simulink model "MOT_CTRL_PWM_FUN_002"  (R2025a)
settings: Solver=FixedStepAuto  StartTime=0.0  StopTime=10.0  FixedStep=1e-4  RelTol=1e-3
settings Model: DataDictionary=PwmGenerator.sldd  Creator=tecnicomcbti  LastModifiedBy=tecnicomcbti

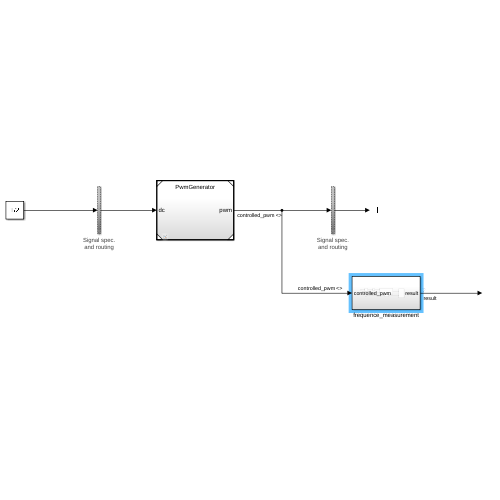
[thumbnail: Simulink's stored preview of the top-level diagram]
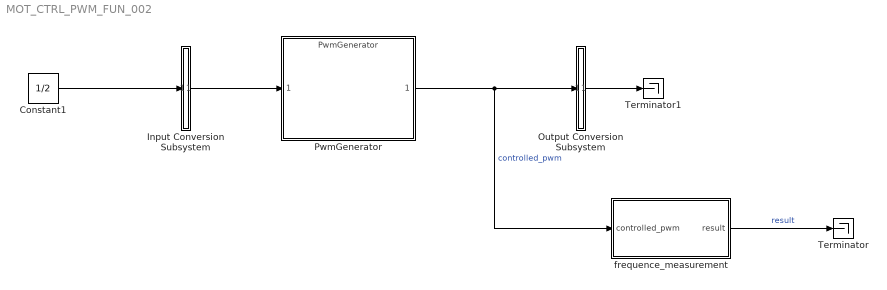
== system MOT_CTRL_PWM_FUN_002 ==
  Constant1 : Constant  Value=1/2
  Input Conversion Subsystem : Subsystem  Tag=__SLT_ICS__  Description=|
      | Signal spec.
      | and routing
      settings: AttributesFormatString=%<Description>
  Output Conversion Subsystem : Subsystem  Tag=__SLT_OCS__  Description=|
      | Signal spec.
      | and routing
      settings: AttributesFormatString=%<Description>
  PwmGenerator : ModelReference  ModelNameDialog=PwmGenerator  SimulationMode=Normal  ModelReferenceVersion=1.9
  Terminator : Terminator
  Terminator1 : Terminator
  frequence_measurement : Subsystem
  wires:
  Constant1/1 -> Input Conversion Subsystem/1(Inport_1)
  Input Conversion Subsystem/1(Outport_1) -> PwmGenerator/1
  PwmGenerator/1 -> frequence_measurement/1(controlled_pwm), Output Conversion Subsystem/1(Inport_1)  "controlled_pwm"
  frequence_measurement/1(result) -> Terminator/1  "result"
  Output Conversion Subsystem/1(Outport_1) -> Terminator1/1

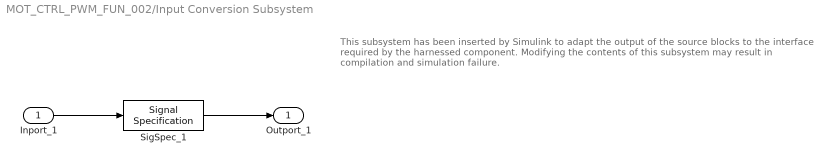
== system MOT_CTRL_PWM_FUN_002/Input Conversion Subsystem ==
  note: This subsystem has been inserted by Simulink to adapt the output of the source blocks to the interface required by the harnessed component.
      |  Modifying the contents of this subsystem may result in compilation and simulation failure.
  Inport_1 : Inport
  SigSpec_1 : SignalSpecification  OutDataTypeStr=double  Dimensions=[1]  SampleTime=0.0001
  Outport_1 : Outport
  wires:
  SigSpec_1/1 -> Outport_1/1
  Inport_1/1 -> SigSpec_1/1

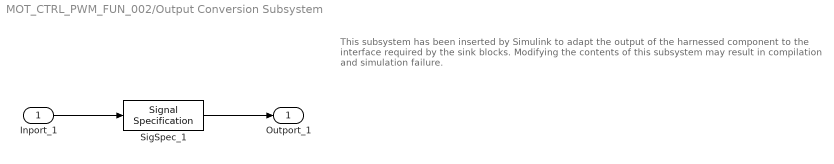
== system MOT_CTRL_PWM_FUN_002/Output Conversion Subsystem ==
  note: This subsystem has been inserted by Simulink to adapt the output of the harnessed component to the interface required by the sink blocks.
      |  Modifying the contents of this subsystem may result in compilation and simulation failure.
  Inport_1 : Inport
  SigSpec_1 : SignalSpecification  OutDataTypeStr=double  Dimensions=[1]  SampleTime=0.0001
  Outport_1 : Outport
  wires:
  Inport_1/1 -> SigSpec_1/1
  SigSpec_1/1 -> Outport_1/1

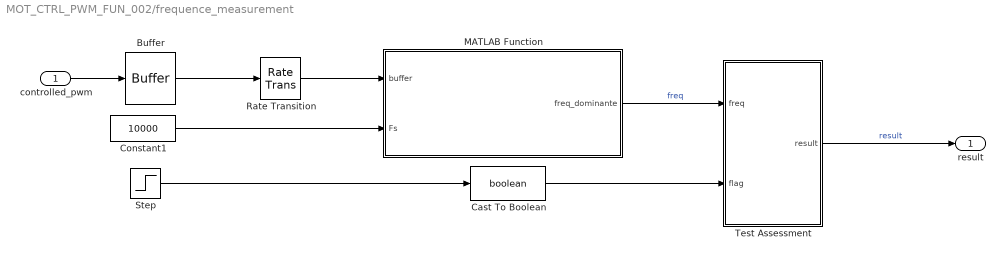
== system MOT_CTRL_PWM_FUN_002/frequence_measurement ==
  controlled_pwm : Inport
  Buffer : Buffer  N=4096  OutputFrames=off
  Cast To Boolean : DataTypeConversion  OutDataTypeStr=boolean  SaturateOnIntegerOverflow=off  RndMeth=Floor
  Constant1 : Constant  Value=10000  SampleTime=1e-4
  MATLAB Function : MATLAB Function  TreatAsAtomicUnit=on
  Rate Transition : RateTransition
  Step : Step  SampleTime=0
  Test Assessment : Test Sequence  TreatAsAtomicUnit=on
  result : Outport
  wires:
  MATLAB Function/1(freq_dominante) -> Test Assessment/1(freq)  "freq"
  Cast To Boolean/1 -> Test Assessment/2(flag)
  Step/1 -> Cast To Boolean/1
  Buffer/1 -> Rate Transition/1
  Test Assessment/1(result) -> result/1  "result"
  Constant1/1 -> MATLAB Function/2(Fs)
  controlled_pwm/1 -> Buffer/1
  Rate Transition/1 -> MATLAB Function/1(buffer)

== stateflow chart MOT_CTRL_PWM_FUN_002/frequence_measurement/Test Assessment ==
  state Test
    if((flag == true) && (freq >= 1000*0.98) && (freq <= 1000*1.02))
    result = true;
    else
    result = false;
    end
  (default) -> Test
  data: freq input; flag input; result output

== matlab function MOT_CTRL_PWM_FUN_002/frequence_measurement/MATLAB Function ==
  data: buffer input; freq_dominante output; Fs input
function freq_dominante = detectarFrequencia(buffer, Fs)
% Calcula a frequência dominante em Hz a partir de um buffer de 4096 amostras
% Entradas:
%   buffer - vetor de 4096 amostras
%   Fs - frequência de amostragem em Hz
% Saída:
%   freq_dominante - frequência dominante em Hz
window_size = 4096;
% Aplica janela de Hamming e remove DC
buffer_processado = buffer .* hamming(window_size);
buffer_processado = buffer_processado - mean(buffer_processado);

% Calcula FFT e obtém magnitude
fft_result = fft(buffer_processado);
magnitude = abs(fft_result(1:window_size/2)); % Metade do espectro

% Encontra o pico ignorando os primeiros bins (DC e baixas frequências)
[~, idx] = max(magnitude(6:end)); % Ignora os 5 primeiros bins
idx = idx + 5; % Ajusta o índice

% Calcula a frequência dominante
freq_dominante = (idx-1) * Fs / window_size;
end
